simulink subsystem "Cubesat_Acceleration"  (R2023a)
settings: Solver=VariableStepAuto  StartTime=0.0  StopTime=10.0  RelTol=1e-3
settings Model: Creator=Andy  LastModifiedBy=Andy

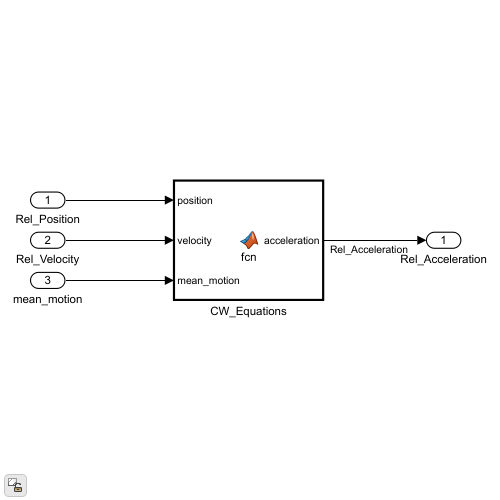
[thumbnail: Simulink's stored preview of the top-level diagram]
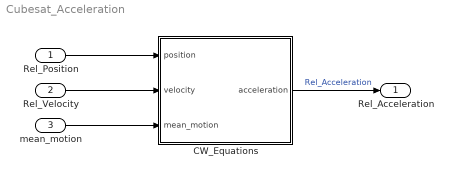
== system Cubesat_Acceleration ==
  Rel_Position : Inport
  Rel_Velocity : Inport  Port=2
  mean_motion : Inport  Port=3
  CW_Equations : MATLAB Function  TreatAsAtomicUnit=on
  Rel_Acceleration : Outport
  wires:
  Rel_Velocity/1 -> CW_Equations/2(velocity)
  CW_Equations/1(acceleration) -> Rel_Acceleration/1  "Rel_Acceleration"
  Rel_Position/1 -> CW_Equations/1(position)
  mean_motion/1 -> CW_Equations/3(mean_motion)

== matlab function Cubesat_Acceleration/CW_Equations ==
  data: position input; acceleration output; velocity input; mean_motion input
function acceleration = fcn(position,velocity,mean_motion)

acceleration = [( 2*mean_motion*velocity(2) + 3*mean_motion^2*position(1)) ...
                 -2*mean_motion*velocity(1) ...
                 -1*mean_motion^2*position(3)];
